simulink model "Copy_of_Trial_86_2"  (R2017b)
settings: Solver=FixedStepDiscrete  StartTime=0.0  StopTime=27  FixedStep=0.01  RelTol=1e-3
libraries: simulink x19
settings Model: Creator=ashwin.ramanujam  LastModifiedBy=gandh
settings DataIOCC: ReturnWorkspaceOutputs=on
settings DebuggingCC: ReadBeforeWriteMsg=DisableAll  WriteAfterWriteMsg=DisableAll  WriteAfterReadMsg=DisableAll  MultiTaskDSMMsg=none
settings ModelReferenceCC: UpdateModelReferenceTargets=IfOutOfDate
settings SFSimCC: SFSimEcho=off

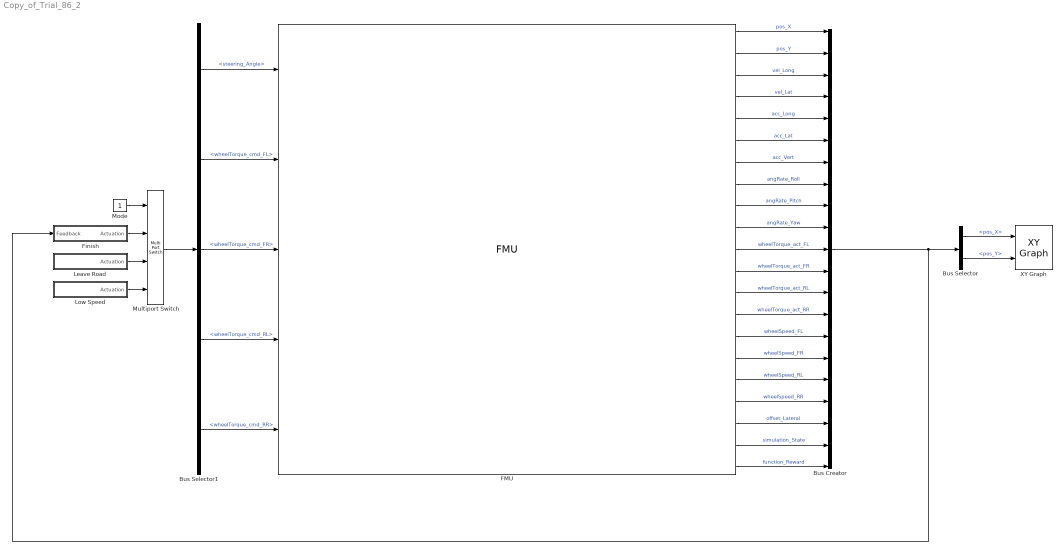
== system Copy_of_Trial_86_2 ==
  Bus Creator : BusCreator  Inputs=21
  Bus Selector : BusSelector  OutputSignals=pos_X,pos_Y
  Bus Selector1 : BusSelector  OutputSignals=steering_Angle,wheelTorque_cmd_FL,wheelTorque_cmd_FR,wheelTorque_cmd_RL,wheelTorque_cmd_RR
  FMU : FMU  FMUName=MED2018_VehicleModel.fmu  FMUDebugLogging=on  FMUMode=CoSimulation  FMUSampleTime=-1  mask(MED2018.VehicleModel [Co-Simulation, v2.0]){}
      mask Display:
      | if (exist([Simulink.fileGenControl('get','CacheFolder') '\slprj\_fmu\d3889ef734f31c902e719d6385a8000b\MED2018_VehicleModel\model.png'],'file'))
      |     image([Simulink.fileGenControl('get','CacheFolder') '\slprj\_fmu\d3889ef734f31c902e719d6385a8000b\MED2018_VehicleModel\model.png']);
      |     text(0.03, 0.97, 'MED2018.VehicleModel', 'horizontalAlignment', 'left', 'verticalAlignment', 'top');
      | else
      |     disp('MED2018.VehicleModel');
      | end
      | port_label('output',1,'pos_X');
      | port_label('output',2,'pos_Y');
      | port_label('output',3,'vel_Long');
      | port_label('output',4,'vel_Lat');
      | port_label('output',5,'acc_Long');
      | port_label('output',6,'acc_Lat');
      | port_label('output',7,'acc_Vert');
      | port_label('output',8,'angRate_Roll');
      | port_label('output',9,'angRate_Pitch');
      | port_label('output',10,'angRate_Yaw');
      | port_label('output',11,'wheellTorque_act_FL');
      | port_label('output',12,'wheelTorque_act_FR');
      | port_label('output',13,'wheelTorque_act_RL');
      | port_label('output',14,'wheelTorque_act_RR');
      | port_label('output',15,'wheelSpeed_FL');
      | port_label('output',16,'wheelSpeed_FR');
      | port_label('output',17,'wheelSpeed_RL');
      | port_label('output',18,'wheelSpeed_RR');
      | port_label('output',19,'offset_Lateral');
      | port_label('output',20,'simulation_State');
      | port_label('output',21,'function_Reward');
      | port_label('input',1,'steering_Angle');
      | port_label('input',2,'wheelTorque_cmd_FL');
      | port_label('input',3,'wheelTorque_cmd_FR');
      | port_label('input',4,'wheelTorque_cmd_RL');
      | port_label('input',5,'wheelTorque_cmd_RR');
  Finish : Subsystem
  Leave Road : Subsystem
  Low Speed : Subsystem
  Mode : Constant
  Multiport Switch : MultiPortSwitch
  XY Graph : simulink/Sinks/XY Graph  xmin=-1  xmax=110  ymin=-10  ymax=180  st=-1
  wires:
  Multiport Switch/1 -> Bus Selector1/1
  Finish/1(Actuation) -> Multiport Switch/2
  Mode/1 -> Multiport Switch/1
  Bus Selector1/1 -> FMU/1  "<steering_Angle>"
  Bus Selector1/2 -> FMU/2  "<wheelTorque_cmd_FL>"
  Bus Selector1/3 -> FMU/3  "<wheelTorque_cmd_FR>"
  Bus Selector1/4 -> FMU/4  "<wheelTorque_cmd_RL>"
  Bus Selector1/5 -> FMU/5  "<wheelTorque_cmd_RR>"
  FMU/1 -> Bus Creator/1  "pos_X"
  FMU/2 -> Bus Creator/2  "pos_Y"
  FMU/3 -> Bus Creator/3  "vel_Long"
  FMU/4 -> Bus Creator/4  "vel_Lat"
  FMU/5 -> Bus Creator/5  "acc_Long"
  FMU/6 -> Bus Creator/6  "acc_Lat"
  FMU/7 -> Bus Creator/7  "acc_Vert"
  FMU/8 -> Bus Creator/8  "angRate_Roll"
  FMU/9 -> Bus Creator/9  "angRate_Pitch"
  FMU/10 -> Bus Creator/10  "angRate_Yaw"
  FMU/11 -> Bus Creator/11  "wheelTorque_act_FL"
  FMU/12 -> Bus Creator/12  "wheelTorque_act_FR"
  FMU/13 -> Bus Creator/13  "wheelTorque_act_RL"
  FMU/14 -> Bus Creator/14  "wheelTorque_act_RR"
  FMU/15 -> Bus Creator/15  "wheelSpeed_FL"
  FMU/16 -> Bus Creator/16  "wheelSpeed_FR"
  FMU/17 -> Bus Creator/17  "wheelSpeed_RL"
  FMU/18 -> Bus Creator/18  "wheelSpeed_RR"
  FMU/19 -> Bus Creator/19  "offset_Lateral"
  FMU/20 -> Bus Creator/20  "simulation_State"
  FMU/21 -> Bus Creator/21  "function_Reward"
  Bus Selector/1 -> XY Graph/1  "<pos_X>"
  Bus Selector/2 -> XY Graph/2  "<pos_Y>"
  Leave Road/1(Actuation) -> Multiport Switch/3
  Low Speed/1(Actuation) -> Multiport Switch/4
  Bus Creator/1 -> Finish/1(Feedback), Bus Selector/1

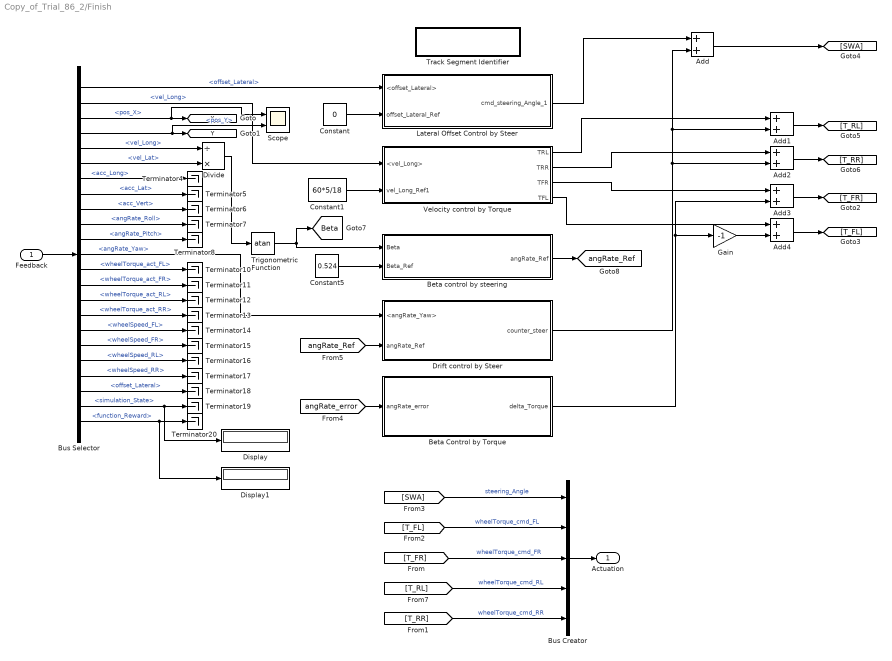
== system Copy_of_Trial_86_2/Finish ==
  Feedback : Inport
  Add{,1..4} (5 alike) : Sum
  Beta Control by Torque : Subsystem
  "Beta control by steering " : Subsystem
  Bus Creator : BusCreator  Inputs=5
  Bus Selector : BusSelector  OutputSignals=offset_Lateral,vel_Long,pos_X,pos_Y,vel_Long,vel_Lat,acc_Long,acc_Lat,acc_Vert,angRate_Roll,angRate_Pitch,angRate_Yaw,wheelTorque_act_FL,wheelTorque_act_FR,wheelTorque_act_RL,wheelTorque_act_RR,wheelSpeed_FL,wheelSpeed_FR,wheelSpeed_RL,wheelSpeed_RR,offset_Lateral,simulation_State,function_Reward
  Constant : Constant  Value=0
  Constant1 : Constant  Value=60*5/18
  Constant5 : Constant  Value=0.524
  Display : Display
  Display1 : Display
  Divide : Product  Inputs=/*
  Drift control by Steer : Subsystem
  Gain : Gain  Gain=-1
  Lateral Offset Control by Steer : Subsystem
  Scope : Scope  NumInputPorts=2
  Terminator{4..8,10..20} (16 alike) : Terminator
  Track Segment Identifier : Subsystem
  Trigonometric Function : Trigonometry  Operator=atan
  Velocity control by Torque : Subsystem
  Actuation : Outport
  tag scope: Beta=global, X=global, Y=global, angRate_Ref=global
  wires:
  Bus Creator/1 -> Actuation/1
  Feedback/1 -> Bus Selector/1
  [T_FL] -> Bus Creator/2  "wheelTorque_cmd_FL"
  [T_RL] -> Bus Creator/4  "wheelTorque_cmd_RL"
  [T_FR] -> Bus Creator/3  "wheelTorque_cmd_FR"
  [T_RR] -> Bus Creator/5  "wheelTorque_cmd_RR"
  Bus Selector/12 -> Drift control by Steer/1(<angRate_Yaw>)  "<angRate_Yaw>"
  Bus Selector/2 -> Velocity control by Torque/1(<vel_Long>)  "<vel_Long>"
  Bus Selector/1 -> Lateral Offset Control by Steer/1(<offset_Lateral>)  "<offset_Lateral>"
  Lateral Offset Control by Steer/1(cmd_steering_Angle_1) -> Add/1
  [SWA] -> Bus Creator/1  "steering_Angle"
  Drift control by Steer/1(counter_steer) -> Add2/2, Add1/2, Add/2
  Bus Selector/4 -> Scope/2, [Y]  "<pos_Y>"
  Bus Selector/3 -> Scope/1, [X]  "<pos_X>"
  Bus Selector/5 -> Divide/1  "<vel_Long>"
  Bus Selector/6 -> Divide/2  "<vel_Lat>"
  Bus Selector/7 -> Terminator4/1  "<acc_Long>"
  Bus Selector/8 -> Terminator5/1  "<acc_Lat>"
  Bus Selector/9 -> Terminator6/1  "<acc_Vert>"
  Bus Selector/10 -> Terminator7/1  "<angRate_Roll>"
  Bus Selector/11 -> Terminator8/1  "<angRate_Pitch>"
  Bus Selector/13 -> Terminator10/1  "<wheelTorque_act_FL>"
  Bus Selector/14 -> Terminator11/1  "<wheelTorque_act_FR>"
  Bus Selector/15 -> Terminator12/1  "<wheelTorque_act_RL>"
  Bus Selector/16 -> Terminator13/1  "<wheelTorque_act_RR>"
  Bus Selector/17 -> Terminator14/1  "<wheelSpeed_FL>"
  Bus Selector/18 -> Terminator15/1  "<wheelSpeed_FR>"
  Bus Selector/19 -> Terminator16/1  "<wheelSpeed_RL>"
  Bus Selector/20 -> Terminator17/1  "<wheelSpeed_RR>"
  Bus Selector/21 -> Terminator18/1  "<offset_Lateral>"
  Bus Selector/22 -> Display/1, Terminator19/1  "<simulation_State>"
  Bus Selector/23 -> Display1/1, Terminator20/1  "<function_Reward>"
  Divide/1 -> Trigonometric Function/1
  Add/1 -> [SWA]
  Constant/1 -> Lateral Offset Control by Steer/2(offset_Lateral_Ref)
  Add1/1 -> [T_RL]
  Add2/1 -> [T_RR]
  Add3/1 -> [T_FR]
  Add4/1 -> [T_FL]
  Velocity control by Torque/1(TRL) -> Add1/1
  Velocity control by Torque/2(TRR) -> Add2/1
  Velocity control by Torque/3(TFR) -> Add3/1
  Velocity control by Torque/4(TFL) -> Add4/1
  Trigonometric Function/1 -> [Beta], "Beta control by steering "/1(Beta)
  Constant1/1 -> Velocity control by Torque/2(vel_Long_Ref1)
  Constant5/1 -> "Beta control by steering "/2(Beta_Ref)
  "Beta control by steering "/1(angRate_Ref) -> [angRate_Ref]
  [angRate_error] -> Beta Control by Torque/1(angRate_error)
  [angRate_Ref] -> Drift control by Steer/2(angRate_Ref)
  Beta Control by Torque/1(delta_Torque) -> Gain/1, Add3/2
  Gain/1 -> Add4/2

== system Copy_of_Trial_86_2/Leave Road ==
  Bus Creator : BusCreator  Inputs=5
  Constant{,1..4} (5 alike) : Constant  Value=0
  Actuation : Outport
  wires:
  Constant4/1 -> Bus Creator/5  "wheelTorque_cmd_RR"
  Constant1/1 -> Bus Creator/2  "wheelTorque_cmd_FL"
  Constant3/1 -> Bus Creator/4  "wheelTorque_cmd_RL"
  Constant/1 -> Bus Creator/1  "steering_Angle"
  Constant2/1 -> Bus Creator/3  "wheelTorque_cmd_FR"
  Bus Creator/1 -> Actuation/1

== system Copy_of_Trial_86_2/Low Speed ==
  Bus Creator : BusCreator  Inputs=5
  Constant : Constant  Value=0
  Constant{1..4} (4 alike) : Constant  Value=-500
  Actuation : Outport
  wires:
  Bus Creator/1 -> Actuation/1
  Constant3/1 -> Bus Creator/4  "wheelTorque_cmd_RL"
  Constant1/1 -> Bus Creator/2  "wheelTorque_cmd_FL"
  Constant/1 -> Bus Creator/1  "steering_Angle"
  Constant4/1 -> Bus Creator/5  "wheelTorque_cmd_RR"
  Constant2/1 -> Bus Creator/3  "wheelTorque_cmd_FR"

== system Copy_of_Trial_86_2/Finish/Beta Control by Torque ==
  angRate_error : Inport
  Discrete PID Controller2 : simulink/Continuous/PID Controller  Controller=PID  TimeDomain=Discrete-time  SampleTime=-1  IntegratorMethod=Forward Euler  FilterMethod=Forward Euler  Form=Parallel  UseFilter=off  ControllerParametersSource=internal  P=800  I=0  D=1  N=100  InitialConditionSource=internal  InitialConditionForIntegrator=0  InitialConditionForFilter=0  ExternalReset=none  LimitOutput=off  UpperSaturationLimit=inf  LowerSaturationLimit=-inf  LinearizeAsGain=off  AntiWindupMode=none  Kb=1  TrackingMode=off  Kt=1  PParamMin=[]  PParamMax=[]  IParamMin=[]  IParamMax=[]  DParamMin=[]  DParamMax=[]  NParamMin=[]  NParamMax=[]  KbParamMin=[]  KbParamMax=[]  KtParamMin=[]  KtParamMax=[]  POutMin=[]  POutMax=[]  IOutMin=[]  IOutMax=[]  DOutMin=[]  DOutMax=[]  NOutMin=[]  NOutMax=[]  KbOutMin=[]  KbOutMax=[]  KtOutMin=[]  KtOutMax=[]  IntegratorOutMin=[]  IntegratorOutMax=[]  FilterOutMin=[]  FilterOutMax=[]  SumOutMin=[]  SumOutMax=[]  SumI1OutMin=[]  SumI1OutMax=[]  SumI2OutMin=[]  SumI2OutMax=[]  SumI3OutMin=[]  SumI3OutMax=[]  SumDOutMin=[]  SumDOutMax=[]  SaturationOutMin=[]  SaturationOutMax=[]  IntegratorContinuousStateAttributes=''  IntegratorStateMustResolveToSignalObject=off  IntegratorRTWStateStorageClass=Auto  FilterContinuousStateAttributes=''  FilterStateMustResolveToSignalObject=off  FilterRTWStateStorageClass=Auto  DifferentiatorICPrevScaledInput=0  DifferentiatorOutMin=[]  DifferentiatorOutMax=[]  InitialConditionSetting=State (most efficient)  FilterDiffOutCoefMin=[]  FilterDiffOutCoefMax=[]  SumDenOutMin=[]  SumDenOutMax=[]  SumNumOutMin=[]  SumNumOutMax=[]  ReciprocalOutMin=[]  ReciprocalOutMax=[]  DivideOutMin=[]  DivideOutMax=[]  TunerSelectOption=Transfer Function Based (PID Tuner App)
  delta_Torque : Outport
  wires:
  Discrete PID Controller2/1 -> delta_Torque/1  "delta_torque"
  angRate_error/1 -> Discrete PID Controller2/1

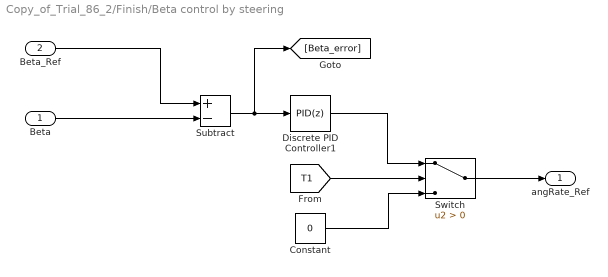
== system Copy_of_Trial_86_2/Finish/Beta control by steering  ==
  Beta : Inport
  Beta_Ref : Inport  Port=2
  Constant : Constant  Value=0
  Discrete PID Controller1 : simulink/Continuous/PID Controller  Controller=PID  TimeDomain=Discrete-time  SampleTime=-1  IntegratorMethod=Forward Euler  FilterMethod=Forward Euler  Form=Parallel  UseFilter=on  ControllerParametersSource=internal  P=1.5  I=0  D=0.1  N=100  InitialConditionSource=internal  InitialConditionForIntegrator=0  InitialConditionForFilter=0  ExternalReset=none  LimitOutput=off  UpperSaturationLimit=inf  LowerSaturationLimit=-inf  LinearizeAsGain=off  AntiWindupMode=none  Kb=1  TrackingMode=off  Kt=1  PParamMin=[]  PParamMax=[]  IParamMin=[]  IParamMax=[]  DParamMin=[]  DParamMax=[]  NParamMin=[]  NParamMax=[]  KbParamMin=[]  KbParamMax=[]  KtParamMin=[]  KtParamMax=[]  POutMin=[]  POutMax=[]  IOutMin=[]  IOutMax=[]  DOutMin=[]  DOutMax=[]  NOutMin=[]  NOutMax=[]  KbOutMin=[]  KbOutMax=[]  KtOutMin=[]  KtOutMax=[]  IntegratorOutMin=[]  IntegratorOutMax=[]  FilterOutMin=[]  FilterOutMax=[]  SumOutMin=[]  SumOutMax=[]  SumI1OutMin=[]  SumI1OutMax=[]  SumI2OutMin=[]  SumI2OutMax=[]  SumI3OutMin=[]  SumI3OutMax=[]  SumDOutMin=[]  SumDOutMax=[]  SaturationOutMin=[]  SaturationOutMax=[]  IntegratorContinuousStateAttributes=''  IntegratorStateMustResolveToSignalObject=off  IntegratorRTWStateStorageClass=Auto  FilterContinuousStateAttributes=''  FilterStateMustResolveToSignalObject=off  FilterRTWStateStorageClass=Auto  DifferentiatorICPrevScaledInput=0  DifferentiatorOutMin=[]  DifferentiatorOutMax=[]  InitialConditionSetting=State (most efficient)  FilterDiffOutCoefMin=[]  FilterDiffOutCoefMax=[]  SumDenOutMin=[]  SumDenOutMax=[]  SumNumOutMin=[]  SumNumOutMax=[]  ReciprocalOutMin=[]  ReciprocalOutMax=[]  DivideOutMin=[]  DivideOutMax=[]  TunerSelectOption=Transfer Function Based (PID Tuner App)
  Subtract : Sum  Inputs=+-
  Switch : Switch  Criteria=u2 > Threshold
  angRate_Ref : Outport
  wires:
  Beta_Ref/1 -> Subtract/1
  Subtract/1 -> [Beta_error], Discrete PID Controller1/1
  Beta/1 -> Subtract/2
  Constant/1 -> Switch/3
  [T1] -> Switch/2
  Switch/1 -> angRate_Ref/1
  Discrete PID Controller1/1 -> Switch/1

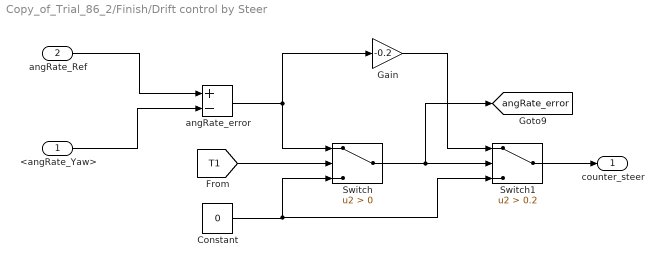
== system Copy_of_Trial_86_2/Finish/Drift control by Steer ==
  <angRate_Yaw> : Inport
  angRate_Ref : Inport  Port=2
  Constant : Constant  Value=0
  Gain : Gain  Gain=-0.2
  Switch : Switch  Criteria=u2 > Threshold
  Switch1 : Switch  Criteria=u2 > Threshold  Threshold=0.2
  angRate_error : Sum  Inputs=+-
  counter_steer : Outport
  tag scope: angRate_error=global
  wires:
  angRate_Ref/1 -> angRate_error/1
  <angRate_Yaw>/1 -> angRate_error/2
  Constant/1 -> Switch1/3, Switch/3
  [T1] -> Switch/2
  Switch/1 -> [angRate_error], Switch1/2
  Switch1/1 -> counter_steer/1
  angRate_error/1 -> Gain/1, Switch/1
  Gain/1 -> Switch1/1

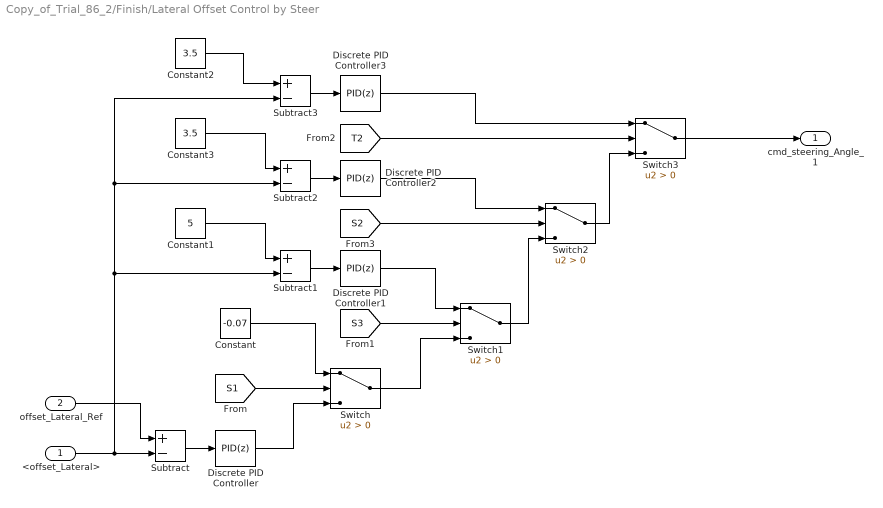
== system Copy_of_Trial_86_2/Finish/Lateral Offset Control by Steer ==
  <offset_Lateral> : Inport
  offset_Lateral_Ref : Inport  Port=2
  Constant : Constant  Value=-0.07
  Constant1 : Constant  Value=5
  Constant2 : Constant  Value=3.5
  Constant3 : Constant  Value=3.5
  Discrete PID Controller : simulink/Continuous/PID Controller  Controller=PID  TimeDomain=Discrete-time  SampleTime=-1  IntegratorMethod=Forward Euler  FilterMethod=Forward Euler  Form=Parallel  UseFilter=off  ControllerParametersSource=internal  P=1  I=0  D=1  N=100  InitialConditionSource=internal  InitialConditionForIntegrator=0  InitialConditionForFilter=0  ExternalReset=none  LimitOutput=off  UpperSaturationLimit=inf  LowerSaturationLimit=-inf  LinearizeAsGain=off  AntiWindupMode=none  Kb=1  TrackingMode=off  Kt=1  PParamMin=[]  PParamMax=[]  IParamMin=[]  IParamMax=[]  DParamMin=[]  DParamMax=[]  NParamMin=[]  NParamMax=[]  KbParamMin=[]  KbParamMax=[]  KtParamMin=[]  KtParamMax=[]  POutMin=[]  POutMax=[]  IOutMin=[]  IOutMax=[]  DOutMin=[]  DOutMax=[]  NOutMin=[]  NOutMax=[]  KbOutMin=[]  KbOutMax=[]  KtOutMin=[]  KtOutMax=[]  IntegratorOutMin=[]  IntegratorOutMax=[]  FilterOutMin=[]  FilterOutMax=[]  SumOutMin=[]  SumOutMax=[]  SumI1OutMin=[]  SumI1OutMax=[]  SumI2OutMin=[]  SumI2OutMax=[]  SumI3OutMin=[]  SumI3OutMax=[]  SumDOutMin=[]  SumDOutMax=[]  SaturationOutMin=[]  SaturationOutMax=[]  IntegratorContinuousStateAttributes=''  IntegratorStateMustResolveToSignalObject=off  IntegratorRTWStateStorageClass=Auto  FilterContinuousStateAttributes=''  FilterStateMustResolveToSignalObject=off  FilterRTWStateStorageClass=Auto  DifferentiatorICPrevScaledInput=0  DifferentiatorOutMin=[]  DifferentiatorOutMax=[]  InitialConditionSetting=State (most efficient)  FilterDiffOutCoefMin=[]  FilterDiffOutCoefMax=[]  SumDenOutMin=[]  SumDenOutMax=[]  SumNumOutMin=[]  SumNumOutMax=[]  ReciprocalOutMin=[]  ReciprocalOutMax=[]  DivideOutMin=[]  DivideOutMax=[]  TunerSelectOption=Transfer Function Based (PID Tuner App)
  Discrete PID Controller1 : simulink/Continuous/PID Controller  Controller=PID  TimeDomain=Discrete-time  SampleTime=-1  IntegratorMethod=Forward Euler  FilterMethod=Forward Euler  Form=Parallel  UseFilter=off  ControllerParametersSource=internal  P=1  I=0  D=1  N=100  InitialConditionSource=internal  InitialConditionForIntegrator=0  InitialConditionForFilter=0  ExternalReset=none  LimitOutput=off  UpperSaturationLimit=inf  LowerSaturationLimit=-inf  LinearizeAsGain=off  AntiWindupMode=none  Kb=1  TrackingMode=off  Kt=1  PParamMin=[]  PParamMax=[]  IParamMin=[]  IParamMax=[]  DParamMin=[]  DParamMax=[]  NParamMin=[]  NParamMax=[]  KbParamMin=[]  KbParamMax=[]  KtParamMin=[]  KtParamMax=[]  POutMin=[]  POutMax=[]  IOutMin=[]  IOutMax=[]  DOutMin=[]  DOutMax=[]  NOutMin=[]  NOutMax=[]  KbOutMin=[]  KbOutMax=[]  KtOutMin=[]  KtOutMax=[]  IntegratorOutMin=[]  IntegratorOutMax=[]  FilterOutMin=[]  FilterOutMax=[]  SumOutMin=[]  SumOutMax=[]  SumI1OutMin=[]  SumI1OutMax=[]  SumI2OutMin=[]  SumI2OutMax=[]  SumI3OutMin=[]  SumI3OutMax=[]  SumDOutMin=[]  SumDOutMax=[]  SaturationOutMin=[]  SaturationOutMax=[]  IntegratorContinuousStateAttributes=''  IntegratorStateMustResolveToSignalObject=off  IntegratorRTWStateStorageClass=Auto  FilterContinuousStateAttributes=''  FilterStateMustResolveToSignalObject=off  FilterRTWStateStorageClass=Auto  DifferentiatorICPrevScaledInput=0  DifferentiatorOutMin=[]  DifferentiatorOutMax=[]  InitialConditionSetting=State (most efficient)  FilterDiffOutCoefMin=[]  FilterDiffOutCoefMax=[]  SumDenOutMin=[]  SumDenOutMax=[]  SumNumOutMin=[]  SumNumOutMax=[]  ReciprocalOutMin=[]  ReciprocalOutMax=[]  DivideOutMin=[]  DivideOutMax=[]  TunerSelectOption=Transfer Function Based (PID Tuner App)
  Discrete PID Controller2 : simulink/Continuous/PID Controller  Controller=PID  TimeDomain=Discrete-time  SampleTime=-1  IntegratorMethod=Forward Euler  FilterMethod=Forward Euler  Form=Parallel  UseFilter=off  ControllerParametersSource=internal  P=1.4  I=0  D=1  N=100  InitialConditionSource=internal  InitialConditionForIntegrator=0  InitialConditionForFilter=0  ExternalReset=none  LimitOutput=off  UpperSaturationLimit=inf  LowerSaturationLimit=-inf  LinearizeAsGain=off  AntiWindupMode=none  Kb=1  TrackingMode=off  Kt=1  PParamMin=[]  PParamMax=[]  IParamMin=[]  IParamMax=[]  DParamMin=[]  DParamMax=[]  NParamMin=[]  NParamMax=[]  KbParamMin=[]  KbParamMax=[]  KtParamMin=[]  KtParamMax=[]  POutMin=[]  POutMax=[]  IOutMin=[]  IOutMax=[]  DOutMin=[]  DOutMax=[]  NOutMin=[]  NOutMax=[]  KbOutMin=[]  KbOutMax=[]  KtOutMin=[]  KtOutMax=[]  IntegratorOutMin=[]  IntegratorOutMax=[]  FilterOutMin=[]  FilterOutMax=[]  SumOutMin=[]  SumOutMax=[]  SumI1OutMin=[]  SumI1OutMax=[]  SumI2OutMin=[]  SumI2OutMax=[]  SumI3OutMin=[]  SumI3OutMax=[]  SumDOutMin=[]  SumDOutMax=[]  SaturationOutMin=[]  SaturationOutMax=[]  IntegratorContinuousStateAttributes=''  IntegratorStateMustResolveToSignalObject=off  IntegratorRTWStateStorageClass=Auto  FilterContinuousStateAttributes=''  FilterStateMustResolveToSignalObject=off  FilterRTWStateStorageClass=Auto  DifferentiatorICPrevScaledInput=0  DifferentiatorOutMin=[]  DifferentiatorOutMax=[]  InitialConditionSetting=State (most efficient)  FilterDiffOutCoefMin=[]  FilterDiffOutCoefMax=[]  SumDenOutMin=[]  SumDenOutMax=[]  SumNumOutMin=[]  SumNumOutMax=[]  ReciprocalOutMin=[]  ReciprocalOutMax=[]  DivideOutMin=[]  DivideOutMax=[]  TunerSelectOption=Transfer Function Based (PID Tuner App)
  Discrete PID Controller3 : simulink/Continuous/PID Controller  Controller=PID  TimeDomain=Discrete-time  SampleTime=-1  IntegratorMethod=Forward Euler  FilterMethod=Forward Euler  Form=Parallel  UseFilter=off  ControllerParametersSource=internal  P=0.9  I=0  D=1  N=100  InitialConditionSource=internal  InitialConditionForIntegrator=0  InitialConditionForFilter=0  ExternalReset=none  LimitOutput=off  UpperSaturationLimit=inf  LowerSaturationLimit=-inf  LinearizeAsGain=off  AntiWindupMode=none  Kb=1  TrackingMode=off  Kt=1  PParamMin=[]  PParamMax=[]  IParamMin=[]  IParamMax=[]  DParamMin=[]  DParamMax=[]  NParamMin=[]  NParamMax=[]  KbParamMin=[]  KbParamMax=[]  KtParamMin=[]  KtParamMax=[]  POutMin=[]  POutMax=[]  IOutMin=[]  IOutMax=[]  DOutMin=[]  DOutMax=[]  NOutMin=[]  NOutMax=[]  KbOutMin=[]  KbOutMax=[]  KtOutMin=[]  KtOutMax=[]  IntegratorOutMin=[]  IntegratorOutMax=[]  FilterOutMin=[]  FilterOutMax=[]  SumOutMin=[]  SumOutMax=[]  SumI1OutMin=[]  SumI1OutMax=[]  SumI2OutMin=[]  SumI2OutMax=[]  SumI3OutMin=[]  SumI3OutMax=[]  SumDOutMin=[]  SumDOutMax=[]  SaturationOutMin=[]  SaturationOutMax=[]  IntegratorContinuousStateAttributes=''  IntegratorStateMustResolveToSignalObject=off  IntegratorRTWStateStorageClass=Auto  FilterContinuousStateAttributes=''  FilterStateMustResolveToSignalObject=off  FilterRTWStateStorageClass=Auto  DifferentiatorICPrevScaledInput=0  DifferentiatorOutMin=[]  DifferentiatorOutMax=[]  InitialConditionSetting=State (most efficient)  FilterDiffOutCoefMin=[]  FilterDiffOutCoefMax=[]  SumDenOutMin=[]  SumDenOutMax=[]  SumNumOutMin=[]  SumNumOutMax=[]  ReciprocalOutMin=[]  ReciprocalOutMax=[]  DivideOutMin=[]  DivideOutMax=[]  TunerSelectOption=Transfer Function Based (PID Tuner App)
  Subtract{,1..3} (4 alike) : Sum  Inputs=+-
  Switch{,1..3} (4 alike) : Switch  Criteria=u2 > Threshold
  cmd_steering_Angle_1 : Outport
  wires:
  offset_Lateral_Ref/1 -> Subtract/1
  Subtract/1 -> Discrete PID Controller/1
  Discrete PID Controller/1 -> Switch/3
  Constant/1 -> Switch/1
  [S1] -> Switch/2
  [S3] -> Switch1/2
  Switch/1 -> Switch1/3
  Discrete PID Controller1/1 -> Switch1/1
  Subtract1/1 -> Discrete PID Controller1/1
  Constant1/1 -> Subtract1/1
  Constant3/1 -> Subtract2/1
  Subtract2/1 -> Discrete PID Controller2/1
  Discrete PID Controller2/1 -> Switch2/1
  Switch1/1 -> Switch2/3
  [S2] -> Switch2/2
  [T2] -> Switch3/2
  Switch3/1 -> cmd_steering_Angle_1/1
  Discrete PID Controller3/1 -> Switch3/1
  Subtract3/1 -> Discrete PID Controller3/1
  <offset_Lateral>/1 -> Subtract2/2, Subtract3/2, Subtract1/2, Subtract/2
  Switch2/1 -> Switch3/3
  Constant2/1 -> Subtract3/1

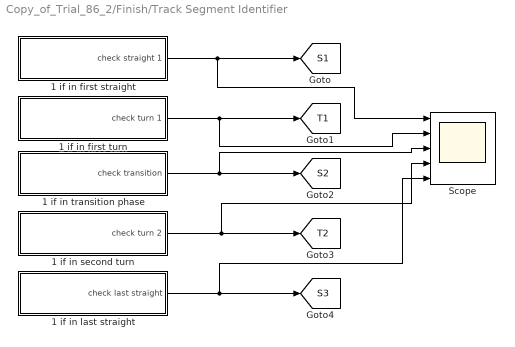
== system Copy_of_Trial_86_2/Finish/Track Segment Identifier ==
  1 if in first straight : Subsystem
  1 if in first turn : Subsystem
  1 if in last straight : Subsystem
  1 if in second turn : Subsystem
  1 if in transition phase : Subsystem
  Scope : Scope  NumInputPorts=5
  tag scope: S1=global, S2=global, S3=global, T1=global, T2=global
  wires:
  1 if in first turn/1(check turn 1) -> Scope/2, [T1]
  1 if in transition phase/1(check transition) -> Scope/3, [S2]
  1 if in first straight/1(check straight 1) -> Scope/1, [S1]
  1 if in second turn/1(check turn 2) -> Scope/4, [T2]
  1 if in last straight/1(check last straight) -> [S3], Scope/5

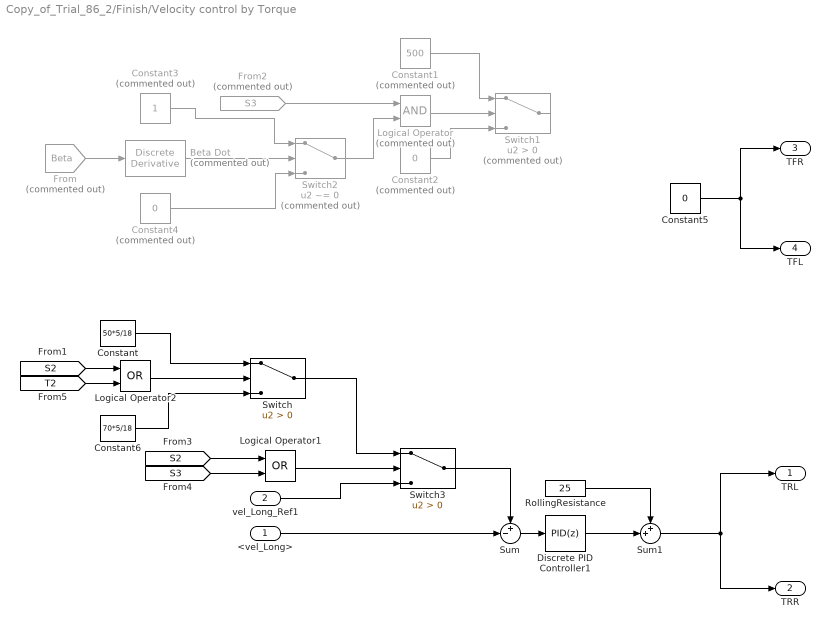
== system Copy_of_Trial_86_2/Finish/Velocity control by Torque ==
  <vel_Long> : Inport
  vel_Long_Ref1 : Inport  Port=2
  Beta Dot : simulink/Discrete/Discrete Derivative  Commented=on  gainval=1.0  ICPrevScaledInput=0.0  OutMin=[]  OutMax=[]  OutDataType=fixdt(1, 16)  OutScaling=2^-10  DoSatur=off
  Constant : Constant  Value=50*5/18
  Constant1 : Constant  Commented=on  Value=500
  Constant2 : Constant  Commented=on  Value=0
  Constant3 : Constant  Commented=on
  Constant4 : Constant  Commented=on  Value=0
  Constant5 : Constant  Value=0
  Constant6 : Constant  Value=70*5/18
  Discrete PID Controller1 : simulink/Continuous/PID Controller  Controller=PID  TimeDomain=Discrete-time  SampleTime=-1  IntegratorMethod=Forward Euler  FilterMethod=Forward Euler  Form=Parallel  UseFilter=on  ControllerParametersSource=internal  P=100  I=0  D=0.1  N=100  InitialConditionSource=internal  InitialConditionForIntegrator=0  InitialConditionForFilter=0  ExternalReset=none  LimitOutput=off  UpperSaturationLimit=inf  LowerSaturationLimit=-inf  LinearizeAsGain=off  AntiWindupMode=none  Kb=1  TrackingMode=off  Kt=1  PParamMin=[]  PParamMax=[]  IParamMin=[]  IParamMax=[]  DParamMin=[]  DParamMax=[]  NParamMin=[]  NParamMax=[]  KbParamMin=[]  KbParamMax=[]  KtParamMin=[]  KtParamMax=[]  POutMin=[]  POutMax=[]  IOutMin=[]  IOutMax=[]  DOutMin=[]  DOutMax=[]  NOutMin=[]  NOutMax=[]  KbOutMin=[]  KbOutMax=[]  KtOutMin=[]  KtOutMax=[]  IntegratorOutMin=[]  IntegratorOutMax=[]  FilterOutMin=[]  FilterOutMax=[]  SumOutMin=[]  SumOutMax=[]  SumI1OutMin=[]  SumI1OutMax=[]  SumI2OutMin=[]  SumI2OutMax=[]  SumI3OutMin=[]  SumI3OutMax=[]  SumDOutMin=[]  SumDOutMax=[]  SaturationOutMin=[]  SaturationOutMax=[]  IntegratorContinuousStateAttributes=''  IntegratorStateMustResolveToSignalObject=off  IntegratorRTWStateStorageClass=Auto  FilterContinuousStateAttributes=''  FilterStateMustResolveToSignalObject=off  FilterRTWStateStorageClass=Auto  DifferentiatorICPrevScaledInput=0  DifferentiatorOutMin=[]  DifferentiatorOutMax=[]  InitialConditionSetting=State (most efficient)  FilterDiffOutCoefMin=[]  FilterDiffOutCoefMax=[]  SumDenOutMin=[]  SumDenOutMax=[]  SumNumOutMin=[]  SumNumOutMax=[]  ReciprocalOutMin=[]  ReciprocalOutMax=[]  DivideOutMin=[]  DivideOutMax=[]  TunerSelectOption=Transfer Function Based (PID Tuner App)
  From : From  Commented=on  GotoTag=Beta  TagVisibility=global
  From2 : From  Commented=on  GotoTag=S3  TagVisibility=global
  Logical Operator : Logic  Commented=on  AllPortsSameDT=off  OutDataTypeStr=boolean
  Logical Operator1 : Logic  Operator=OR  AllPortsSameDT=off  OutDataTypeStr=boolean
  Logical Operator2 : Logic  Operator=OR  AllPortsSameDT=off  OutDataTypeStr=boolean
  RollingResistance : Constant  Value=25
  Sum : Sum  Inputs=+-|
  Sum1 : Sum  Inputs=++|
  Switch : Switch  Criteria=u2 > Threshold
  Switch1 : Switch  Commented=on  Criteria=u2 > Threshold
  Switch2 : Switch  Commented=on  Criteria=u2 ~= 0
  Switch3 : Switch  Criteria=u2 > Threshold
  TRL : Outport
  TRR : Outport  Port=2
  TFR : Outport  Port=3
  TFL : Outport  Port=4
  wires:
  RollingResistance/1 -> Sum1/1
  <vel_Long>/1 -> Sum/2
  Sum/1 -> Discrete PID Controller1/1
  Discrete PID Controller1/1 -> Sum1/2
  Constant2/1 -> Switch1/3
  Constant1/1 -> Switch1/1
  From2/1 -> Logical Operator/1
  From/1 -> Beta Dot/1
  Logical Operator/1 -> Switch1/2
  Switch2/1 -> Logical Operator/2
  Beta Dot/1 -> Switch2/2
  Constant3/1 -> Switch2/1
  Constant4/1 -> Switch2/3
  Sum1/1 -> TRL/1, TRR/1
  Constant/1 -> Switch/1
  Constant6/1 -> Switch/3
  vel_Long_Ref1/1 -> Switch3/3
  Switch3/1 -> Sum/1
  Logical Operator1/1 -> Switch3/2
  Switch/1 -> Switch3/1
  [S3] -> Logical Operator1/2
  [S2] -> Logical Operator1/1
  Logical Operator2/1 -> Switch/2
  [S2] -> Logical Operator2/1
  [T2] -> Logical Operator2/2
  Constant5/1 -> TFL/1, TFR/1

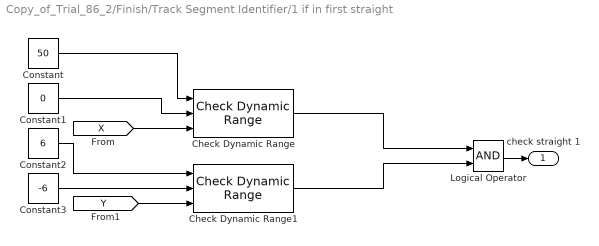
== system Copy_of_Trial_86_2/Finish/Track Segment Identifier/1 if in first straight ==
  Check Dynamic Range : simulink/Model Verification/Check  Dynamic Range  Description=min < u < max  enabled=off  stopWhenAssertionFail=off  export=on  icon=graphic
      settings: SourceProductName=Simulink  SourceProductBaseCode=SL
  Check Dynamic Range1 : simulink/Model Verification/Check  Dynamic Range  Description=min < u < max  enabled=off  stopWhenAssertionFail=off  export=on  icon=graphic
      settings: SourceProductName=Simulink  SourceProductBaseCode=SL
  Constant : Constant  Value=50
  Constant1 : Constant  Value=0
  Constant2 : Constant  Value=6
  Constant3 : Constant  Value=-6
  Logical Operator : Logic  AllPortsSameDT=off  OutDataTypeStr=boolean
  check straight 1 : Outport
  wires:
  [Y] -> Check Dynamic Range1/3
  Check Dynamic Range1/1 -> Logical Operator/2
  Constant1/1 -> Check Dynamic Range/2
  [X] -> Check Dynamic Range/3
  Check Dynamic Range/1 -> Logical Operator/1
  Constant3/1 -> Check Dynamic Range1/2
  Constant2/1 -> Check Dynamic Range1/1
  Logical Operator/1 -> check straight 1/1
  Constant/1 -> Check Dynamic Range/1

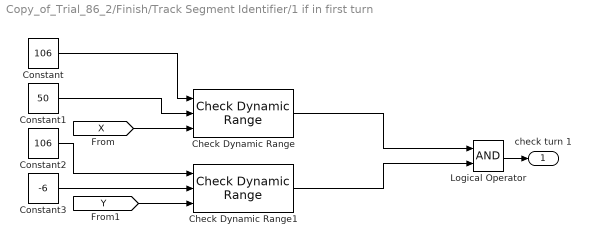
== system Copy_of_Trial_86_2/Finish/Track Segment Identifier/1 if in first turn ==
  Check Dynamic Range : simulink/Model Verification/Check  Dynamic Range  Description=min < u < max  enabled=off  stopWhenAssertionFail=off  export=on  icon=graphic
      settings: SourceProductName=Simulink  SourceProductBaseCode=SL
  Check Dynamic Range1 : simulink/Model Verification/Check  Dynamic Range  Description=min < u < max  enabled=off  stopWhenAssertionFail=off  export=on  icon=graphic
      settings: SourceProductName=Simulink  SourceProductBaseCode=SL
  Constant : Constant  Value=106
  Constant1 : Constant  Value=50
  Constant2 : Constant  Value=106
  Constant3 : Constant  Value=-6
  Logical Operator : Logic  AllPortsSameDT=off  OutDataTypeStr=boolean
  check turn 1 : Outport
  wires:
  Constant/1 -> Check Dynamic Range/1
  Logical Operator/1 -> check turn 1/1
  Constant2/1 -> Check Dynamic Range1/1
  Constant3/1 -> Check Dynamic Range1/2
  Check Dynamic Range/1 -> Logical Operator/1
  [X] -> Check Dynamic Range/3
  Constant1/1 -> Check Dynamic Range/2
  Check Dynamic Range1/1 -> Logical Operator/2
  [Y] -> Check Dynamic Range1/3

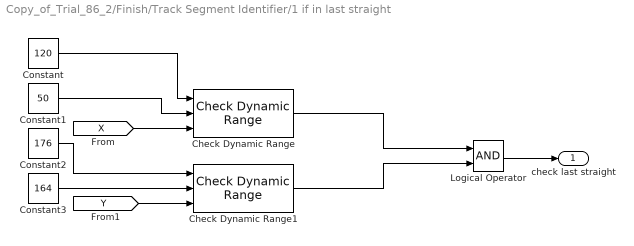
== system Copy_of_Trial_86_2/Finish/Track Segment Identifier/1 if in last straight ==
  Check Dynamic Range : simulink/Model Verification/Check  Dynamic Range  Description=min < u < max  enabled=off  stopWhenAssertionFail=off  export=on  icon=graphic
      settings: SourceProductName=Simulink  SourceProductBaseCode=SL
  Check Dynamic Range1 : simulink/Model Verification/Check  Dynamic Range  Description=min < u < max  enabled=off  stopWhenAssertionFail=off  export=on  icon=graphic
      settings: SourceProductName=Simulink  SourceProductBaseCode=SL
  Constant : Constant  Value=120
  Constant1 : Constant  Value=50
  Constant2 : Constant  Value=176
  Constant3 : Constant  Value=164
  Logical Operator : Logic  AllPortsSameDT=off  OutDataTypeStr=boolean
  check last straight : Outport
  wires:
  [Y] -> Check Dynamic Range1/3
  Check Dynamic Range1/1 -> Logical Operator/2
  Constant1/1 -> Check Dynamic Range/2
  [X] -> Check Dynamic Range/3
  Check Dynamic Range/1 -> Logical Operator/1
  Constant3/1 -> Check Dynamic Range1/2
  Constant2/1 -> Check Dynamic Range1/1
  Logical Operator/1 -> check last straight/1
  Constant/1 -> Check Dynamic Range/1

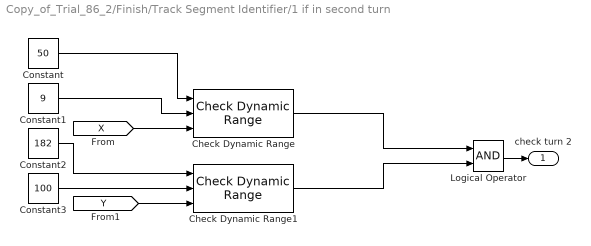
== system Copy_of_Trial_86_2/Finish/Track Segment Identifier/1 if in second turn ==
  Check Dynamic Range : simulink/Model Verification/Check  Dynamic Range  Description=min < u < max  enabled=off  stopWhenAssertionFail=off  export=on  icon=graphic
      settings: SourceProductName=Simulink  SourceProductBaseCode=SL
  Check Dynamic Range1 : simulink/Model Verification/Check  Dynamic Range  Description=min < u < max  enabled=off  stopWhenAssertionFail=off  export=on  icon=graphic
      settings: SourceProductName=Simulink  SourceProductBaseCode=SL
  Constant : Constant  Value=50
  Constant1 : Constant  Value=9
  Constant2 : Constant  Value=182
  Constant3 : Constant  Value=100
  Logical Operator : Logic  AllPortsSameDT=off  OutDataTypeStr=boolean
  check turn 2 : Outport
  wires:
  Constant/1 -> Check Dynamic Range/1
  Logical Operator/1 -> check turn 2/1
  Constant2/1 -> Check Dynamic Range1/1
  Constant3/1 -> Check Dynamic Range1/2
  Check Dynamic Range/1 -> Logical Operator/1
  [X] -> Check Dynamic Range/3
  Constant1/1 -> Check Dynamic Range/2
  Check Dynamic Range1/1 -> Logical Operator/2
  [Y] -> Check Dynamic Range1/3

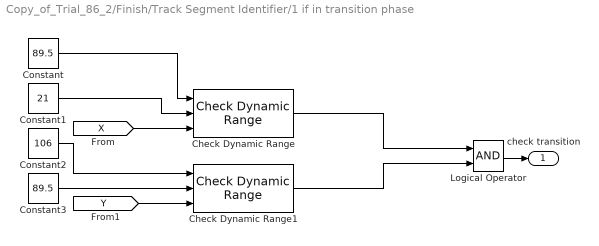
== system Copy_of_Trial_86_2/Finish/Track Segment Identifier/1 if in transition phase ==
  Check Dynamic Range : simulink/Model Verification/Check  Dynamic Range  Description=min < u < max  enabled=off  stopWhenAssertionFail=off  export=on  icon=graphic
      settings: SourceProductName=Simulink  SourceProductBaseCode=SL
  Check Dynamic Range1 : simulink/Model Verification/Check  Dynamic Range  Description=min < u < max  enabled=off  stopWhenAssertionFail=off  export=on  icon=graphic
      settings: SourceProductName=Simulink  SourceProductBaseCode=SL
  Constant : Constant  Value=89.5
  Constant1 : Constant  Value=21
  Constant2 : Constant  Value=106
  Constant3 : Constant  Value=89.5
  Logical Operator : Logic  AllPortsSameDT=off  OutDataTypeStr=boolean
  check transition : Outport
  wires:
  [Y] -> Check Dynamic Range1/3
  Check Dynamic Range1/1 -> Logical Operator/2
  Constant1/1 -> Check Dynamic Range/2
  [X] -> Check Dynamic Range/3
  Check Dynamic Range/1 -> Logical Operator/1
  Constant3/1 -> Check Dynamic Range1/2
  Constant2/1 -> Check Dynamic Range1/1
  Logical Operator/1 -> check transition/1
  Constant/1 -> Check Dynamic Range/1
